simulink model "new_algorithm"  (R2023b)
settings: Solver=VariableStepAuto  StartTime=0.0  StopTime=10.0  RelTol=1e-3
libraries: dspadpt3 x1, audiosources x1
settings Model: Creator=mykni  LastModifiedBy=mykni

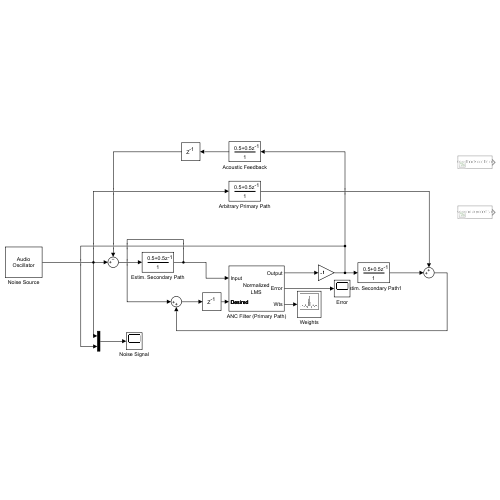
[thumbnail: Simulink's stored preview of the top-level diagram]
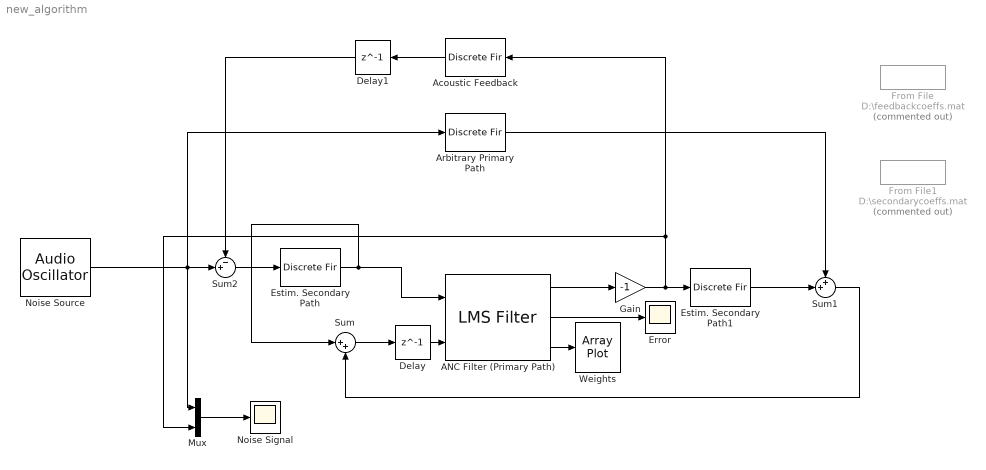
== system new_algorithm ==
  ANC Filter (Primary Path) : dspadpt3/LMS Filter  Algo=Normalized LMS  L=32  stepflag=Dialog  mu=.005  leakage=1.0  ic=0  Adapt=off  resetflag=None  weights=on  addnparflag=off  roundingMode=Floor  overflowMode=off
  Acoustic Feedback : DiscreteFir
  Arbitrary Primary Path : DiscreteFir
  Delay : Delay  DelayLength=1  InitialCondition=0
  Delay1 : Delay  DelayLength=1  InitialCondition=0
  Error : Scope
  Estim. Secondary Path : DiscreteFir
  Estim. Secondary Path1 : DiscreteFir
  From File : FromFile  Commented=on  FileName=D:\feedbackcoeffs.mat  SampleTime=0
  From File1 : FromFile  Commented=on  FileName=D:\secondarycoeffs.mat  SampleTime=0
  Gain : Gain  Gain=-1
  Mux : Mux  Inputs=2
  Noise Signal : Scope
  Noise Source : audiosources/Audio Oscillator  FrequencyPort=off  Frequency=100  AmplitudePort=off  Amplitude=1  DCOffsetPort=off  PhaseOffset=0  DCOffset=0  WidthPort=off  Width=1  DutyCyclePort=off  DutyCycle=0.5  SampsPerFrame=10  Fs=44100  OutputDataType=double  SimulateUsing=Code generation
      settings: SignalType=sine
  Sum : Sum  Inputs=|++
  Sum1 : Sum  Inputs=++|
  Sum2 : Sum  Inputs=-+|
  Weights : ArrayPlot  WindowPosition=[368.000000,182.000000,800.000000,500.000000,]  ScopeFrameLocation=window  YLimits=[-0.0551 0.1188]
  wires:
  Noise Source/1 -> Mux/1, Sum2/2, Arbitrary Primary Path/1
  Estim. Secondary Path/1 -> Sum/1, ANC Filter (Primary Path)/1
  ANC Filter (Primary Path)/1 -> Gain/1
  Gain/1 -> Acoustic Feedback/1, Mux/2, Estim. Secondary Path1/1
  Estim. Secondary Path1/1 -> Sum1/2
  Sum1/1 -> Sum/2
  Arbitrary Primary Path/1 -> Sum1/1
  ANC Filter (Primary Path)/2 -> Error/1
  ANC Filter (Primary Path)/3 -> Weights/1
  Sum/1 -> Delay/1
  Delay/1 -> ANC Filter (Primary Path)/2
  Mux/1 -> Noise Signal/1
  Acoustic Feedback/1 -> Delay1/1
  Delay1/1 -> Sum2/1
  Sum2/1 -> Estim. Secondary Path/1
